simulink model "PID_tp4"  (R2024b)
settings: Solver=VariableStepAuto  StartTime=0.0  RelTol=1e-3
values from neighbouring files (symbols this model uses):
  perturbance_time_apply = 10*Lp    (= 57)    [resolucion_matlab.m]
  step_time_apply = 1    [resolucion_matlab.m]
libraries: cstblocks x2
settings Model: Creator=tomii  LastModifiedBy=tomii

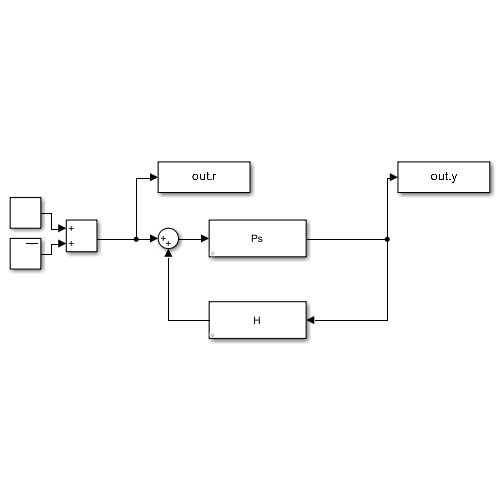
[thumbnail: Simulink's stored preview of the top-level diagram]
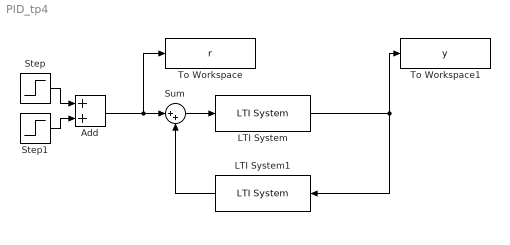
== system PID_tp4 ==
  Add : Sum
  LTI System : cstblocks/LTI System  sys=Ps  IC=[]  PadeOrder=0
  LTI System1 : cstblocks/LTI System  sys=H  IC=[]  PadeOrder=0
  Step : Step  Time=step_time_apply  SampleTime=0
  Step1 : Step  Time=perturbance_time_apply  After=0.2  SampleTime=0
  Sum : Sum  Inputs=|++
  To Workspace : ToWorkspace  VariableName=r  SaveFormat=Timeseries  SampleTime=-1
  To Workspace1 : ToWorkspace  VariableName=y  SaveFormat=Timeseries  SampleTime=-1
  wires:
  Sum/1 -> LTI System/1
  Step/1 -> Add/1
  Step1/1 -> Add/2
  Add/1 -> To Workspace/1, Sum/1
  LTI System/1 -> To Workspace1/1, LTI System1/1
  LTI System1/1 -> Sum/2
